simulink model "MMFA"  (R2020b)
settings: Solver=VariableStepAuto  StartTime=0.0  StopTime=inf  RelTol=1e-3
libraries: commutil2 x9, dspfdesign x8
settings Model: Creator=fernando  LastModifiedBy=fernando
settings DebuggingCC: UnderSpecifiedDimensionMsg=warning

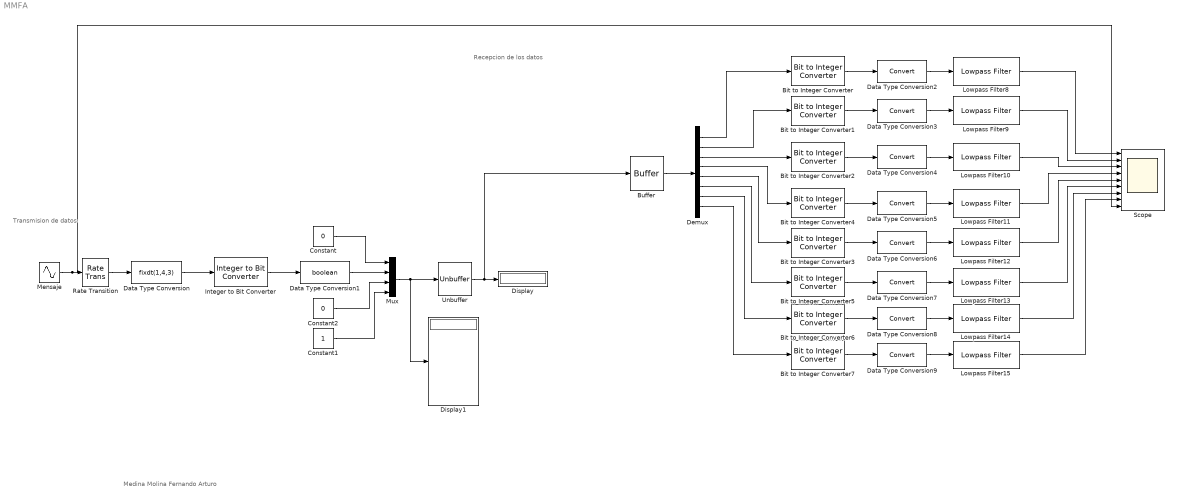
== system MMFA ==
  note: Recepcion de los datos
  note: Transmision de datos
  note: Medina Molina Fernando Arturo
  Bit to Integer Converter{,1..7} (8 alike) : commutil2/Bit to Integer Converter  nbits=8  bitOrder=MSB first  signedOutputValues=Unsigned  outDtype=Inherit via internal rule  outDtypeSigned=Inherit via internal rule
  Buffer : Buffer  OutputFrames=off
  Constant : Constant  Value=0  OutDataTypeStr=boolean
  Constant1 : Constant  OutDataTypeStr=boolean
  Constant2 : Constant  Value=0  OutDataTypeStr=boolean
  Data Type Conversion : DataTypeConversion  OutDataTypeStr=fixdt(1,4,3)
  Data Type Conversion1 : DataTypeConversion  OutDataTypeStr=boolean
  Data Type Conversion{2..9} (8 alike) : DataTypeConversion
  Demux : Demux  Outputs=8
  Display : Display
  Display1 : Display
  Integer to Bit Converter : commutil2/Integer to Bit Converter  nbits=4  signedInputValues=Unsigned  bitOrder=MSB first  outDtype=Inherit via internal rule
  Lowpass Filter{8..15} (8 alike) : dspfdesign/Lowpass Filter  FilterType=FIR  DesignForMinimumOrder=on  FilterOrder=50  PassbandFrequency=8e3  StopbandFrequency=12e3  PassbandRipple=0.1  StopbandAttenuation=80  InheritSampleRate=off  SampleRate=44100  SimulateUsing=Interpreted execution  roundingMode=Floor  coeffsDataTypeStr=fixdt(1,16)
  Mensaje : Sin  Frequency=2*pi*400  SampleTime=0
  Mux : Mux
  Rate Transition : RateTransition  OutPortSampleTime=1/4000
  Scope : Scope  NumInputPorts=9
  Unbuffer : Unbuffer
  wires:
  Mensaje/1 -> Scope/9, Rate Transition/1
  Rate Transition/1 -> Data Type Conversion/1
  Data Type Conversion/1 -> Integer to Bit Converter/1
  Unbuffer/1 -> Buffer/1, Display/1
  Constant/1 -> Mux/1
  Constant2/1 -> Mux/3
  Constant1/1 -> Mux/4
  Mux/1 -> Display1/1, Unbuffer/1
  Integer to Bit Converter/1 -> Data Type Conversion1/1
  Data Type Conversion1/1 -> Mux/2
  Buffer/1 -> Demux/1
  Demux/2 -> Bit to Integer Converter1/1
  Demux/3 -> Bit to Integer Converter2/1
  Demux/4 -> Bit to Integer Converter4/1
  Demux/5 -> Bit to Integer Converter3/1
  Demux/6 -> Bit to Integer Converter5/1
  Demux/7 -> Bit to Integer Converter6/1
  Demux/8 -> Bit to Integer Converter7/1
  Bit to Integer Converter7/1 -> Data Type Conversion9/1
  Bit to Integer Converter6/1 -> Data Type Conversion8/1
  Bit to Integer Converter/1 -> Data Type Conversion2/1
  Bit to Integer Converter1/1 -> Data Type Conversion3/1
  Bit to Integer Converter2/1 -> Data Type Conversion4/1
  Bit to Integer Converter4/1 -> Data Type Conversion5/1
  Bit to Integer Converter3/1 -> Data Type Conversion6/1
  Bit to Integer Converter5/1 -> Data Type Conversion7/1
  Data Type Conversion2/1 -> Lowpass Filter8/1
  Data Type Conversion3/1 -> Lowpass Filter9/1
  Data Type Conversion4/1 -> Lowpass Filter10/1
  Data Type Conversion5/1 -> Lowpass Filter11/1
  Data Type Conversion6/1 -> Lowpass Filter12/1
  Data Type Conversion7/1 -> Lowpass Filter13/1
  Data Type Conversion8/1 -> Lowpass Filter14/1
  Data Type Conversion9/1 -> Lowpass Filter15/1
  Lowpass Filter8/1 -> Scope/1
  Lowpass Filter9/1 -> Scope/2
  Lowpass Filter10/1 -> Scope/3
  Lowpass Filter11/1 -> Scope/4
  Lowpass Filter12/1 -> Scope/5
  Lowpass Filter13/1 -> Scope/6
  Lowpass Filter14/1 -> Scope/7
  Lowpass Filter15/1 -> Scope/8
  Demux/1 -> Bit to Integer Converter/1
